simulink model "mpt_demo_rtw_onlinempc"  (Simulink 7.9)
settings: Solver=FixedStepDiscrete  StartTime=0.0  StopTime=10.0  RelTol=1e-3
values from neighbouring files (symbols this model uses):
  problem = Opt(v.constraints,v.objective,theta,[inputs(:); states(:); outputs(:)])    [mpt_demo_deployment_onlineMPC.m]
settings Model: Creator=mato  LastModifiedBy=machine
settings HardwareCC: ProdIntDivRoundTo=Zero  ProdEndianess=LittleEndian  ProdHWDeviceType=Generic->32-bit x86 compatible
settings RTWCC: SystemTargetFile=rtwin.tlc  TemplateMakefile=lcp_rtwin.tmf  Description=Real-Time Windows Target  ProcessScript=rtwin_make_rtw_hook  CustomInclude="\"C:\\mpt\\mpt_devel\\tbxmanager\\toolboxes\\lcprtw\\1.0\\pcwin\\lcp_rtw2012a\\lib\" \"C:\\mpt\\mpt_devel\\tbxmanager\\toolboxes\\lcp\\1.0.2\\pcwin\\source\""  CustomSource=lcp_main.c lcp_matrix.c lumod_dense.c  CustomLibrary=lcp_rtwin.lib  RTWCompilerOptimization=On
settings CodeAppCC: MaxIdLength=95
settings RTWinTargetCC: TargetLibSuffix=_rtwin.lib  TargetPreCompLibLocation=C:\Program Files\MATLAB\R2012a\toolbox\rtw\targets\rtwin\lib\win32  CodeReplacementLibrary=ANSI_C  CodeExecutionProfiling=off  PortableWordSizes=off  RTWinDir=C:/PROGRA~1/MATLAB/R2012a/toolbox/rtw/targets/rtwin  TargetArch=win32

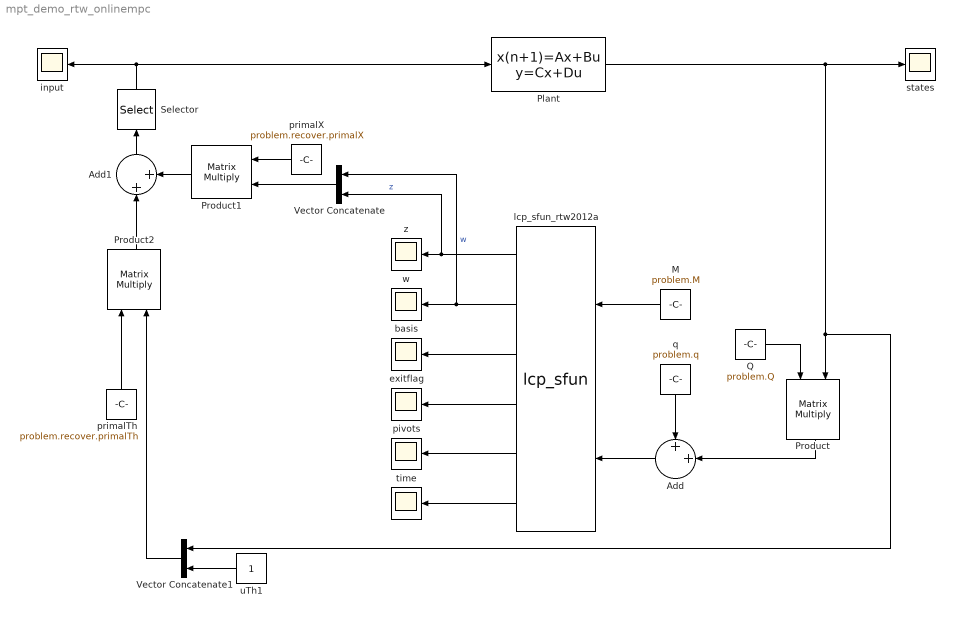
== system mpt_demo_rtw_onlinempc ==
  Add : Sum  Inputs=++|
  Add1 : Sum  Inputs=|++
  M : Constant  Value=problem.M
  Plant : DiscreteStateSpace  A="[0.5403   -0.8415; 0.8415    0.5403]"  B=[ -0.4597; 0.8415]  C=eye(2)  D=[0;0]  X0=[-2;3]
  Product : Product  Multiplication=Matrix(*)  RndMeth=Zero
  Product1 : Product  Multiplication=Matrix(*)  RndMeth=Zero
  Product2 : Product  Multiplication=Matrix(*)  RndMeth=Zero
  Q : Constant  Value=problem.Q
  Selector : Selector  InputPortWidth=20  IndexOptions=Index vector (dialog)  Indices=[1]  OutputSizes=1
  Vector Concatenate : Concatenate
  Vector Concatenate1 : Concatenate
  basis : Scope
      settings: SaveName=ScopeData2
  exitflag : Scope
      settings: SaveName=ScopeData3
  input : Scope
  lcp_sfun_rtw2012a : S-Function  FunctionName=lcp_sfun  Parameters=n,ts  EnableBusSupport=off  mask(LCP solver){n=problem.n, ts=1}
      mask prompts: n "Number of variables in LCP"; ts "Sampling time"
      mask help: Linear-complementarity problem (LCP) solver.
      mask init:
      | % find where LCP solver is installed
      | p = which('lcp');
      | 
      | if isempty(p)
      |     error('Could not find path to LCP solver. Add LCP solver to Matlab path.');
      | end
      | 
      | if ispc
      |     % find where RTW templates are installed
      |     s = which('lcp_rtwin.tmf');
      |     if isempty(s)
      |         error('Could not find RTW templates for LCP solver. Add the path to the LCP solver configured for for Real-Time Workshop "lcprtw" or install it using tbxmanager.');
      |     end
      |     
      |     lib_path = ['"',fileparts(s),filesep,'lib" '];
      |     src_path = ['"',fileparts(p),'" '];
      |     
      |     % set path to external libs
      |     set_param(strtok(gcs,'/'),'CustomInclude',[lib_path,src_path]);
      |     
      |     % set sources
      |     set_param(strtok(gcs,'/'),'CustomSource','lcp_main.c lcp_matrix.c lumod_dense.c ');
      |     
      |     % what is the target ?
      |     target = get_param(strtok(gcs,'/'),'SystemTargetFile');
      |     
      |     if strcmp(target,'rtwin.tlc')
      |         
      |         % set LCP template
      |         try
      |             set_param(strtok(gcs,'/'),'TemplateMakefile','lcp_rtwin.tmf');
      |         catch
      |             msgbox('LCP initialization script have changed the default settings, try to compile the scheme again with "CTRL+B".');
      |             set_param(strtok(gcs,'/'),'TemplateMakefile','lcp_rtwin.tmf');
      |         end
      |         % set libs
      |         set_param(strtok(gcs,'/'),'CustomLibrary','lcp_rtwin.lib');
      |         
      |     elseif strcmp(target,'xpctarget.tlc')
      |         
      |         % check for OpenWatcom compiler
      |         if ~strcmpi(getxpcenv('CCompiler'),'Watcom')
      |             error('You need to set OpenWatcom compiler for XPC target to work with LCP. You can download the compiler from "www.openwatcom.org".');
      |         end
      |         
      |         % set LCP template
      |         try
      |             set_param(strtok(gcs,'/'),'TemplateMakefile','lcp_xpc_watc.tmf');
      |         catch
      |             msgbox('LCP initialization script have changed the default settings, try to compile the scheme again with "CTRL+B".');
      |             set_param(strtok(gcs,'/'),'TemplateMakefile','lcp_xpc_watc.tmf');
      |         end
      |         % set libs
      |         set_param(strtok(gcs,'/'),'CustomLibrary','lcp_mex.lib flib7s.lib');
      |         
      |     elseif strcmp(target,'grt.tlc')
      |         
      |         % check for a compiler
      |         cn = mex.getCompilerConfigurations;
      |         
      |         % set libs
      |         if ~isempty(regexpi(cn(1).Name,'microsoft'))
      |             dirstr='microsoft';
      |             libs = [matlabroot,filesep,'extern',filesep,'lib',filesep,'win32',filesep,dirstr,filesep];
      |             
      |             % set default template
      |             try
      |                 set_param(strtok(gcs,'/'),'TemplateMakefile','grt_default_tmf');
      |                 set_param(strtok(gcs,'/'),'CustomLibrary',['"',libs,'libmwblas.lib" "',libs,'libmwlapack.lib"']);
      |             catch
      |                 msgbox('LCP initialization script have changed the default settings, try to compile the scheme again with "CTRL+B".');
      |                 set_param(strtok(gcs,'/'),'TemplateMakefile','grt_default_tmf');
      |                 set_param(strtok(gcs,'/'),'CustomLibrary',['"',libs,'libmwblas.lib" "',libs,'libmwlapack.lib"']);
      |             end
      |             
      |         elseif ~isempty(regexpi(cn(1).Name,'watcom'))
      |             
      |             % set LCP template
      |             try
      |                 set_param(strtok(gcs,'/'),'TemplateMakefile','lcp_grt_watc.tmf');
      |                 set_param(strtok(gcs,'/'),'CustomLibrary','lcp_mex.lib flib7s.lib');
      |             catch
      |                 msgbox('LCP initialization script have changed the default settings, try to compile the scheme again with "CTRL+B".');
      |                 set_param(strtok(gcs,'/'),'TemplateMakefile','lcp_grt_watc.tmf');
      |                 set_param(strtok(gcs,'/'),'CustomLibrary','lcp_mex.lib flib7s.lib');
      |             end
      |             
      |         elseif ~isempty(regexpi(cn(1).Name,'lcc'))
      |             dirstr='lcc';
      |             libs = [matlabroot,filesep,'extern',filesep,'lib',filesep,'win32',filesep,dirstr,filesep];
      |             
      |             % set default template
      |             try
      |                 set_param(strtok(gcs,'/'),'TemplateMakefile','grt_default_tmf');
      |                 set_param(strtok(gcs,'/'),'CustomLibrary',['"',libs,'libmwblas.lib" "',libs,'libmwlapack.lib"']);
      |             catch
      |                 msgbox('LCP initialization script have changed the default settings, try to compile the scheme again with "CTRL+B".');
      |                 set_param(strtok(gcs,'/'),'TemplateMakefile','grt_default_tmf');
      |                 set_param(strtok(gcs,'/'),'CustomLibrary',['"',libs,'libmwblas.lib" "',libs,'libmwlapack.lib"']);
      |             end
      |             
      |         else
      |             error('You don''t have a suitable C-compiler installed.');
      |         end
      |         
      |         
      |     else
      |         if ~isempty(which('rtwbuild'))
      |             disp(' ');
      |             disp('============================================================================');
      |             fprintf('This target for Real-Time Workshop has not been tested with LCP solver,\nyou may experience problems when compiling, linking and running.\nPlease, choose RTWIN or XPC target.\n');
      |             fprintf('Alternatively, you can recompile the source fils for this target\non your own. The source files are located in "openwatcom/DBLAS_DLAPAC_SRC" directory.\n');
      |             disp('============================================================================');
      |             disp(' ');
      |         end
      |     end
      | end
      mask Help:
      | <pre>
      | LCP: Matlab interface to lexicographic Lemke algorithm
      | =======================================================
      | 
      | 
      | SYNTAX
      | ------
      | 
      |     [z, w, basis, exitflag, pivots, time] = lcp(M, q, options)
      | 
      | 
      | DESCRIPTION
      | -----------
      |    The lexicographic Lemke algorithm solves linear-complementarity problem (LCP) of the form
      |                                           find   w, z            (1)
      |                                           s.t.   w - Mz = q      (2)
      |                                                  w >= 0          (3)
      |                                                  z >= 0          (4)
      |                                                 w'*z = 0         (5)
      | 
      |   where w, z  are the unknown variables, and M, q  are given. For a feasible solution, matrix M
      |   should be positive-semidefinite. The complentarity condition w'z=0 ensures that either one, or both
      |   elements of vectors w, z  are zero.
      | 
      | INPUT
      | -----
      | 
      | 
      |     M                 positive semi-definite square patrix (for a
      |                       feasible solution)
      |                       Class: double
      |     q                 right hand side vector with dimension equal M
      |                       Class: double
      |     options           options structure
      |                       Class: struct
      |     options.zerotol   Less than this treshold the value is considered as
      |                       zero.
      |                       Class: double
      |                       Default: 1e-10
      |     options.lextol    Lexicographic tolerance - a small treshold from
      |                       which values are considered as equal.
      |                       Class: double
      |                       Default: 1e-10
      |     options.maxpiv    Maximum number of pivots to be performed.
      |                       Class: double
      |                       Default: 1e6
      |     options.nstepf    If routine is 0, then every 50 pivot steps the
      |                       basis is refactorized to avoid numerical problems
      |                       for LUMOD. For other routines the factorization is
      |                       performed at each step.
      |                       Class: double
      |                       Default: 50
      |     options.clock     Show the information about the computational time.
      | 
      |                       Class: double
      |                       Allowed values:
      | 
      |                         0
      |                         1
      | 
      |                       Default: 0
      |     options.verbose   Verbose output. Show progress of pivoting
      |                       algorithm including entering, leaving variables,
      |                       actual basis and basis solution.
      |                       Class: double
      |                       Allowed values:
      | 
      |                         0
      |                         1
      | 
      |                       Default: 0
      |     options.routine   Routine which should be used to obtain a basis
      |                       solution.
      |                       Class: double
      |                       Allowed values:
      | 
      |                         0  Corresponds to LUmod package that performs
      |                          factorization in the form LA = U. Depending on
      |                          the change in A  factors L, U  are updated.
      |                          This is the fastest method.
      |                         1  Corresponds to DGESV simple driver from
      |                          LAPACK package which solves the system AX = B
      |                          by factorizing A and overwriting B with the
      |                          solution X. Since the factorization is
      |                          performed at each pivot step, this method tends
      |                          to be much slower than method 0.
      |                         2  Corresponds to DGELS simple driver which
      |                          solves overdetermined or underdetermined real
      |                          linear systems min ||b - Ax||_2 involving an
      |                          M-by- N  matrix A, or its transpose, using a QR
      |                          or LQ factorization of A. Since the
      |                          factorization is performed at each pivot step,
      |                          this method tends to be much slower than method
      |                          0.
      | 
      |                       Default: 0
      |     options.timelimit Time limit in seconds. If this limit is exceeded,
      |                       the pivoting algorithm is terminated and current
      |                       basis is returned.
      |                       Class: double
      |                       Default: 3600
      |     options.normalize Input matrices M, q  get scaled by D1  and
      |                       D2 when invoking this option: Mn = D1M*D2, qn =
      |                       D1*q, and solution is recovered as z = D2*zn, w =
      |                       Mz+q.
      |                       Class: double
      |                       Allowed values:
      | 
      |                         0
      |                         1
      | 
      |                       Default: 1
      | 
      | 
      | 
      | OUTPUT
      | ------
      | 
      | 
      |     z        Solution vector to the linear complementarity
      |              problem
      |              Class: double
      |     w        Complementary vector to z.
      |              Class: double
      |     basis    Index set describing the feasible basis.
      |              Class: double
      |     exitflag Information on how the algorithm terminated.
      |              Class: double
      |              Allowed values:
      | 
      |                1  feasible solution
      |               -1  infeasible
      |               -2  unbounded
      |               -3  preterminated (due to time limit or maximum
      |                   pivot limit )
      |               -4  other (numerical) error
      | 
      |     pivots   Total number of pivots performed by the algorithm.
      |              Class: double
      | 
      |     time     Time needed for algorithm to terminate (in
      |              seconds).
      |              Class: double
      | 
      | 
      | 
      | EXAMPLE(s)
      | ----------
      | 
      | 
      | Example 1
      | =========
      |   % A simple example
      |     M = [1 -1 -1 -1; -1 1 -1 -1; 1 1 2 0; 1 1 0 2]
      |     q = [3, 5, -9, -5]
      |     [z,w,basis,exitflag,pivots] = lcp([1 -1 -1 -1;-1 1 -1 -1; 1 1 2 0;1 1 0 2],[3;5;-9;-5])
      | 
      | 
      | AUTHOR(s)
      | ---------
      | 
      | 
      |  (c) 2010  Colin Neil Jones: ETH Zurich
      |  cjones@control.ee.ethz.ch
      | 
      | 
      |  (c) 2010  Martin Herceg: ETH Zurich
      |   herceg@control.ee.ethz.ch
      | 
      | 
      | LICENSE
      | -------
      | 
      |   This program is free software; you can redistribute it and/or modify it under the terms of the GNU
      | General Public License as published by the Free Software Foundation; either version 2.1 of the
      | License, or (at your option) any later version.
      |   This program is distributed in the hope that it will be useful, but WITHOUT ANY WARRANTY; without
      | even the implied warranty of MERCHANTABILITY or FITNESS FOR A PARTICULAR PURPOSE. See the GNU
      | General Public License for more details.
      |   You should have received a copy of the GNU General Public License along with this library; if not,
      | write to the  Free Software Foundation, Inc.,  59 Temple Place, Suite 330,  Boston, MA 02111-1307
      | USA
      | 
      | </pre>
      mask Display: disp('LCP solver\n for RTW 2012a');
  pivots : Scope
      settings: SaveName=ScopeData4
  primalTh : Constant  Value=problem.recover.primalTh
  primalX : Constant  Value=problem.recover.primalX
  q : Constant  Value=problem.q
  states : Scope
  time : Scope
      settings: SaveName=ScopeData5
  uTh1 : Constant
  w : Scope
      settings: SaveName=ScopeData6
  z : Scope
      settings: SaveName=ScopeData7
  wires:
  Plant/1 -> states/1, Product/2, Vector Concatenate1/1
  lcp_sfun_rtw2012a/1 -> z/1, Vector Concatenate/2  "z"
  M/1 -> lcp_sfun_rtw2012a/1
  lcp_sfun_rtw2012a/2 -> w/1, Vector Concatenate/1  "w"
  lcp_sfun_rtw2012a/3 -> basis/1
  lcp_sfun_rtw2012a/4 -> exitflag/1
  lcp_sfun_rtw2012a/5 -> pivots/1
  lcp_sfun_rtw2012a/6 -> time/1
  Add/1 -> lcp_sfun_rtw2012a/2
  q/1 -> Add/1
  Q/1 -> Product/1
  Product/1 -> Add/2
  primalX/1 -> Product1/1
  Vector Concatenate/1 -> Product1/2
  Product1/1 -> Add1/2
  Product2/1 -> Add1/1
  primalTh/1 -> Product2/1
  Vector Concatenate1/1 -> Product2/2
  uTh1/1 -> Vector Concatenate1/2
  Add1/1 -> Selector/1
  Selector/1 -> input/1, Plant/1
